simulink model "Rudder_system_control2020_5"  (R2022b)
settings: Solver=VariableStepAuto  StartTime=0.0  StopTime=1800  MaxStep=0.02  RelTol=1e-3  AbsTol=1e-3  EnableMultiTasking=on
model workspace (MAT data in the model file):
  lowerLimitSaturation = -0.1
  upperLimitSaturation = 0.1
values from neighbouring files (symbols this model uses):
  Fg = 1    [start.m]
  H = 1    [start.m]
  Js = 1    [start.m]
  PistonStroke = 0.6    [start.m]
undefined symbols (not defined in the file or in its folder): sigbuilder_block
libraries: fl_lib x71, nesl_utility x16, sh_lib x2, simulink x1, aerolibconvert2 x1
(part 2 of 2)

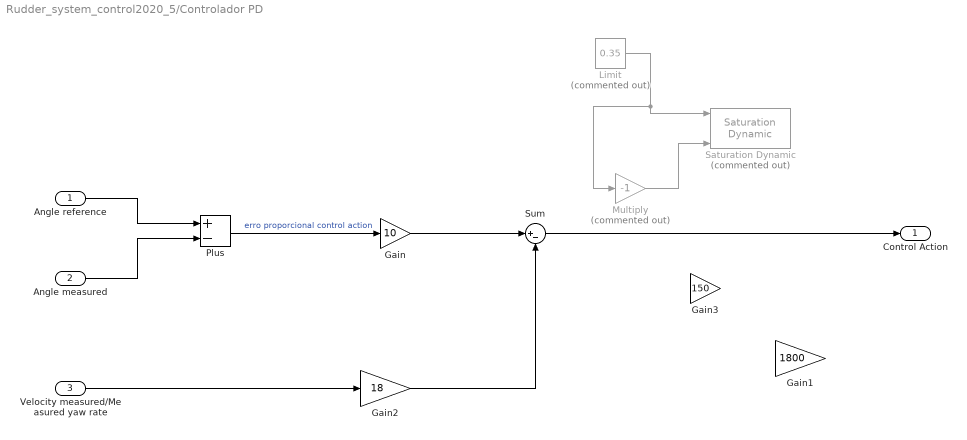
== system Rudder_system_control2020_5/Controlador PD ==
  Angle reference : Inport
  Angle measured : Inport  Port=2
  Velocity measured/Measured yaw rate : Inport  Port=3
  Gain : Gain  Gain=10
  Gain1 : Gain  Gain=1800
  Gain2 : Gain  Gain=18
  Gain3 : Gain  Gain=150
  Limit : Constant  Commented=on  Value=0.35
  Multiply : Gain  Commented=on  Gain=-1
  Plus : Sum  Inputs=+-
  Saturation Dynamic : simulink/Discontinuities/Saturation Dynamic  Commented=on  OutMin=[]  OutMax=[]  OutDataTypeStr=Inherit: Same as second input  OutDataType=fixdt(1, 16)  OutScaling=2^-10  DoSatur=off
  Sum : Sum  Inputs=|+-
  Control Action : Outport
  wires:
  Plus/1 -> Gain/1  "erro proporcional control action"
  Angle reference/1 -> Plus/1
  Angle measured/1 -> Plus/2
  Limit/1 -> Multiply/1, Saturation Dynamic/1
  Multiply/1 -> Saturation Dynamic/3
  Velocity measured/Measured yaw rate/1 -> Gain2/1
  Gain/1 -> Sum/1
  Sum/1 -> Control Action/1
  Gain2/1 -> Sum/2

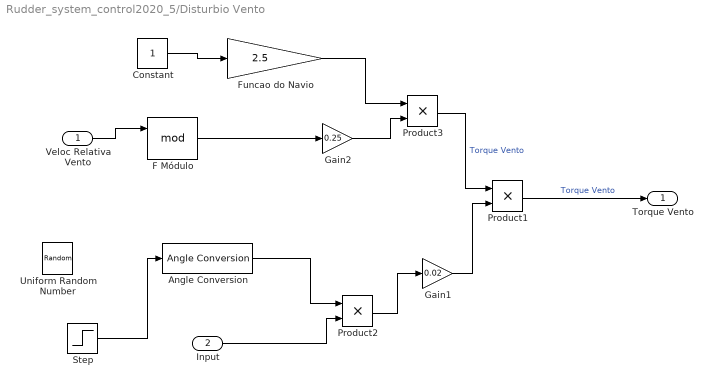
== system Rudder_system_control2020_5/Disturbio Vento ==
  Veloc Relativa Vento : Inport
  Input : Inport  Port=2
  Angle Conversion : aerolibconvert2/Angle Conversion  IU=rad  OU=deg
  Constant : Constant
  F Módulo : Math  Operator=mod
  Funcao do Navio : Gain  Gain=2.5
  Gain1 : Gain  Gain=0.02
  Gain2 : Gain  Gain=0.25
  Product1 : Product
  Product2 : Product
  Product3 : Product
  Step : Step  After=pi*0.5  SampleTime=0
  Uniform Random Number : UniformRandomNumber  Minimum=-2*pi  Maximum=2*pi  SampleTime=30
  Torque Vento : Outport
  wires:
  F Módulo/1 -> Gain2/1
  Gain2/1 -> Product3/2
  Angle Conversion/1 -> Product2/1
  Input/1 -> Product2/2
  Product2/1 -> Gain1/1
  Product1/1 -> Torque Vento/1  "Torque Vento"
  Veloc Relativa Vento/1 -> F Módulo/1
  Funcao do Navio/1 -> Product3/1
  Product3/1 -> Product1/1  "Torque Vento"
  Constant/1 -> Funcao do Navio/1
  Gain1/1 -> Product1/2
  Step/1 -> Angle Conversion/1

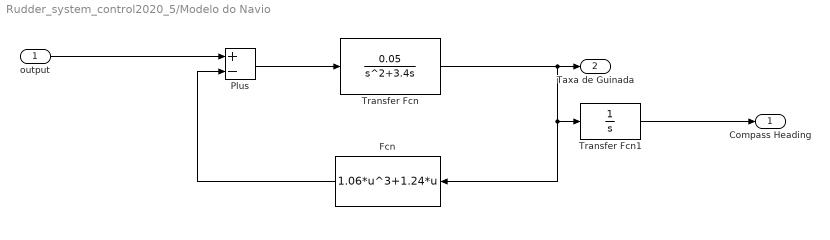
== system Rudder_system_control2020_5/Modelo do Navio ==
  output : Inport
  Fcn : Fcn  Expr=1.06*u^3+1.24*u
  Plus : Sum  Inputs=+-
  Transfer Fcn : TransferFcn  Numerator=[0.05]  Denominator=[1 3.4 0]
  Transfer Fcn1 : TransferFcn  Denominator=[1 0]
  Compass Heading : Outport
  Taxa de Guinada : Outport  Port=2
  wires:
  output/1 -> Plus/1
  Transfer Fcn1/1 -> Compass Heading/1
  Fcn/1 -> Plus/2
  Transfer Fcn/1 -> Fcn/1, Transfer Fcn1/1, Taxa de Guinada/1
  Plus/1 -> Transfer Fcn/1

== system Rudder_system_control2020_5/Signal Builder ==
  Demux : Demux  Tag=STV Demux  Outputs=1
      settings: DisplayOption=none
  FromWs : FromWorkspace  Tag=STV FromWs  VariableName=tuvar
      SigBuilderData=|
      | common.afterFinalStr = 'Extrapolate'
      | common.sampleTime = 0
      | dataSet.timeRange = [0 3000]
      | dataSet.name = 'Group 1'
      | sbobj.Groups.Name = 'Group 1'
      | sbobj.Groups.Signals.Name = 'Signal 2'
      | sbobj.Groups.Signals.XData = [0 10 10 3000]
      | sbobj.Groups.Signals.YData = [0 0 1 1]
      | sbobj.Groups.TimeRange = [0 3000]
  Signal 2 : Outport  Tag=STV Outport
  wires:
  FromWs/1 -> Demux/1
  Demux/1 -> Signal 2/1

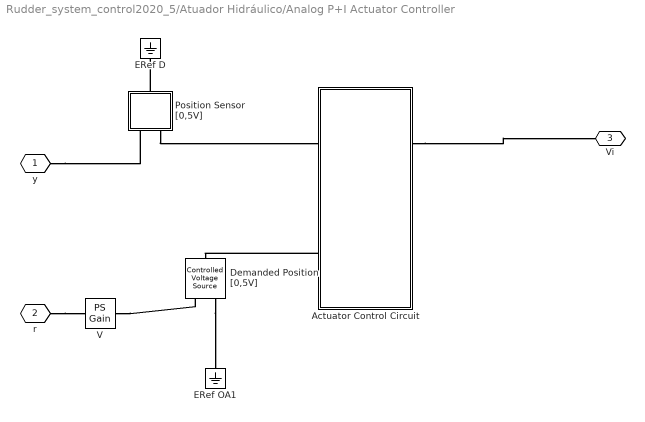
== system Rudder_system_control2020_5/Atuador Hidráulico/Analog P+I Actuator Controller ==
  Actuator Control Circuit : Subsystem  Tag=PublishSubsystem
  Demanded Position [0,5V] : fl_lib/Electrical/Electrical Sources/Controlled Voltage Source
  ERef D : fl_lib/Electrical/Electrical Elements/Electrical Reference
  ERef OA1 : fl_lib/Electrical/Electrical Elements/Electrical Reference
  Position Sensor [0,5V] : Subsystem
  V : fl_lib/Physical Signals/Functions/PS Gain  gain=1 V
  y : PMIOPort  Tag=PMCPort  Side=Left
  r : PMIOPort  Tag=PMCPort  Port=2  Side=Left
  Vi : PMIOPort  Port=3  Side=Right
  connections:
  y/RConn1 -- Position Sensor [0,5V]/LConn1
  r/RConn1 -- V/LConn1
  Actuator Control Circuit/LConn2 -- Demanded Position [0,5V]/LConn1
  Position Sensor [0,5V]/RConn1 -- ERef D/LConn1
  Position Sensor [0,5V]/LConn2 -- Actuator Control Circuit/LConn1
  Actuator Control Circuit/RConn1 -- Vi/RConn1
  Demanded Position [0,5V]/RConn2 -- ERef OA1/LConn1
  V/RConn1 -- Demanded Position [0,5V]/RConn1

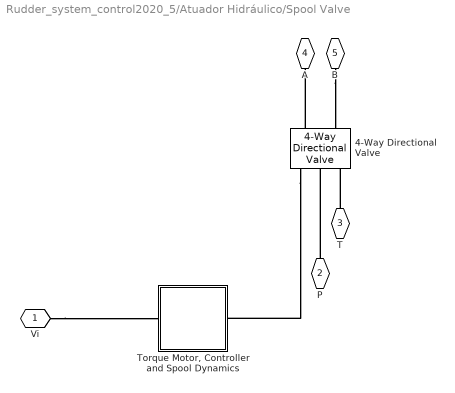
== system Rudder_system_control2020_5/Atuador Hidráulico/Spool Valve ==
  4-Way Directional Valve : sh_lib/Valves/Directional Valves/4-Way Directional Valve  area_spec=sh.valves.directional_valves.enum.area_spec.identical  mdl_type_identical=sh.valves.directional_valves.enum.mdl_type.linear  mdl_type_different=sh.valves.directional_valves.enum.mdl_type.linear  interp_method_identical=sh.valves.directional_valves.enum.interp_method.linear  interp_method_different=sh.valves.directional_valves.enum.interp_method.linear  extrap_method_identical=sh.valves.directional_valves.enum.extrap_method.linear  extrap_method_different=sh.valves.directional_valves.enum.extrap_method.linear  A_leak=1e-12 m^2  C_d=0.7  lam_spec=sh.valves.directional_valves.enum.lam_spec.pressure_ratio  B_lam=0.999  Re_cr=12  opening_max=0.005 m  area_max=0.5e-4 m^2  opening_max_P_A=0.005 m  area_max_P_A=0.5e-4 m^2  opening_max_P_B=0.005 m  area_max_P_B=0.5e-4 m^2  opening_max_A_T=0.005 m  area_max_A_T=0.5e-4 m^2  opening_max_B_T=0.005 m  area_max_B_T=0.5e-4 m^2  opening_area_tab=[-.002, 0, .002, .005, .015] m  area_tab=[1e-09, 2.0352e-07, 4.0736e-05, .00011438, .00034356] m^2  opening_flow_rate_tab=[-.002, 0, .002, .005, .015] m  pressure_tab=[-10000000, -5000000, -2000000, 2000000, 5000000, 10000000] Pa  flow_rate_tab=[-1e-07, -7.0711e-08, -4.4721e-08, 4.4721e-08, 7.0711e-08, 1e-07; -2.0352e-05, -1.4391e-05, -9.1017e-06, 9.1017e-06, 1.4391e-05, 2.0352e-05; -.0040736, -.0028805, -.0018218, .0018218, .0028805, .0040736; -.011438, -.0080879, -.0051152, .0051152, .0080879, .011438; -.034356, -.024293, -.015364, .015364, .024293, .034356] m^3/s  opening_area_tab_P_A=[-.002, 0, .002, .005, .015] m  area_tab_P_A=[1e-09, 2.0352e-07, 4.0736e-05, .00011438, .00034356] m^2  opening_flow_rate_tab_P_A=[-.002, 0, .002, .005, .015] m  pressure_tab_P_A=[-10000000, -5000000, -2000000, 2000000, 5000000, 10000000] Pa  flow_rate_tab_P_A=[-1e-07, -7.0711e-08, -4.4721e-08, 4.4721e-08, 7.0711e-08, 1e-07; -2.0352e-05, -1.4391e-05, -9.1017e-06, 9.1017e-06, 1.4391e-05, 2.0352e-05; -.0040736, -.0028805, -.0018218, .0018218, .0028805, .0040736; -.011438, -.0080879, -.0051152, .0051152, .0080879, .011438; -.034356, -.024293, -.015364, .015364, .024293, .034356] m^3/s  opening_area_tab_P_B=[-.002, 0, .002, .005, .015] m  area_tab_P_B=[1e-09, 2.0352e-07, 4.0736e-05, .00011438, .00034356] m^2  opening_flow_rate_tab_P_B=[-.002, 0, .002, .005, .015] m  pressure_tab_P_B=[-10000000, -5000000, -2000000, 2000000, 5000000, 10000000] Pa  flow_rate_tab_P_B=[-1e-07, -7.0711e-08, -4.4721e-08, 4.4721e-08, 7.0711e-08, 1e-07; -2.0352e-05, -1.4391e-05, -9.1017e-06, 9.1017e-06, 1.4391e-05, 2.0352e-05; -.0040736, -.0028805, -.0018218, .0018218, .0028805, .0040736; -.011438, -.0080879, -.0051152, .0051152, .0080879, .011438; -.034356, -.024293, -.015364, .015364, .024293, .034356] m^3/s  opening_area_tab_A_T=[-.002, 0, .002, .005, .015] m  area_tab_A_T=[1e-09, 2.0352e-07, 4.0736e-05, .00011438, .00034356] m^2  opening_flow_rate_tab_A_T=[-.002, 0, .002, .005, .015] m  pressure_tab_A_T=[-10000000, -5000000, -2000000, 2000000, 5000000, 10000000] Pa  flow_rate_tab_A_T=[-1e-07, -7.0711e-08, -4.4721e-08, 4.4721e-08, 7.0711e-08, 1e-07; -2.0352e-05, -1.4391e-05, -9.1017e-06, 9.1017e-06, 1.4391e-05, 2.0352e-05; -.0040736, -.0028805, -.0018218, .0018218, .0028805, .0040736; -.011438, -.0080879, -.0051152, .0051152, .0080879, .011438; -.034356, -.024293, -.015364, .015364, .024293, .034356] m^3/s  opening_area_tab_B_T=[-.002, 0, .002, .005, .015] m  area_tab_B_T=[1e-09, 2.0352e-07, 4.0736e-05, .00011438, .00034356] m^2  opening_flow_rate_tab_B_T=[-.002, 0, .002, .005, .015] m  pressure_tab_B_T=[-10000000, -5000000, -2000000, 2000000, 5000000, 10000000] Pa  flow_rate_tab_B_T=[-1e-07, -7.0711e-08, -4.4721e-08, 4.4721e-08, 7.0711e-08, 1e-07; -2.0352e-05, -1.4391e-05, -9.1017e-06, 9.1017e-06, 1.4391e-05, 2.0352e-05; -.0040736, -.0028805, -.0018218, .0018218, .0028805, .0040736; -.011438, -.0080879, -.0051152, .0051152, .0080879, .011438; -.034356, -.024293, -.015364, .015364, .024293, .034356] m^3/s  x_0_P_A=0 m  x_0_P_B=0 m  x_0_A_T=0 m  x_0_B_T=0 m
      settings: InternalSimscapePortConfiguration="{\"Bottom\":[],\"Left\":[{\"id\":\"A\",\"label\":\"A\",\"type\":\"foundation.hydraulic.hydraulic\"},{\"id\":\"B\",\"label\":\"B\",\"type\":\"foundation.hydraulic.hydraulic\"}],\"Right\":[{\"id\":\"S\",\"label\":\"S\",\"type\":\"input\"},{\"id\":\"P\",\"label\":\"P\",\"type\":\"foundation.hydraulic.hydraulic\"},{\"id\":\"T\",\"label\":\"T\",\"type\":\"foundation.hydraulic.hydraulic\"}],\"Top\":[]}"
  "Torque Motor, Controller and Spool Dynamics" : Subsystem
  Vi : PMIOPort  Tag=PMCPort  Side=Left
  P : PMIOPort  Tag=PMCPort  Port=2  Side=Left
  T : PMIOPort  Tag=PMCPort  Port=3  Side=Left
  A : PMIOPort  Tag=PMCPort  Port=4  Side=Right
  B : PMIOPort  Tag=PMCPort  Port=5  Side=Right
  connections:
  Vi/RConn1 -- "Torque Motor, Controller and Spool Dynamics"/LConn1
  4-Way Directional Valve/RConn1 -- "Torque Motor, Controller and Spool Dynamics"/RConn1
  4-Way Directional Valve/LConn1 -- A/RConn1
  B/RConn1 -- 4-Way Directional Valve/LConn2
  P/RConn1 -- 4-Way Directional Valve/RConn2
  T/RConn1 -- 4-Way Directional Valve/RConn3

== system Rudder_system_control2020_5/Atuador Hidráulico/Supply Pressure ==
  Supply Pressure : Constant  Value=200
  bar : nesl_utility/Simulink-PS Converter  PhysicalDomain=network_engine_domain  SubClassName=ps_input  LeftPortType=input  RightPortType=output  PseudoPeriodic=off  Frequencies=[]  NoiseDistribution=none  NoiseParameters=[]  Unit=bar  AffineConversion=off  FilteringAndDerivatives=zero  SimscapeFilterOrder=1  InputFilterTimeConstant=.001  UdotUserProvided=0
  S : PMIOPort  Side=Right
  wires:
  Supply Pressure/1 -> bar/1
  connections:
  bar/RConn1 -- S/RConn1

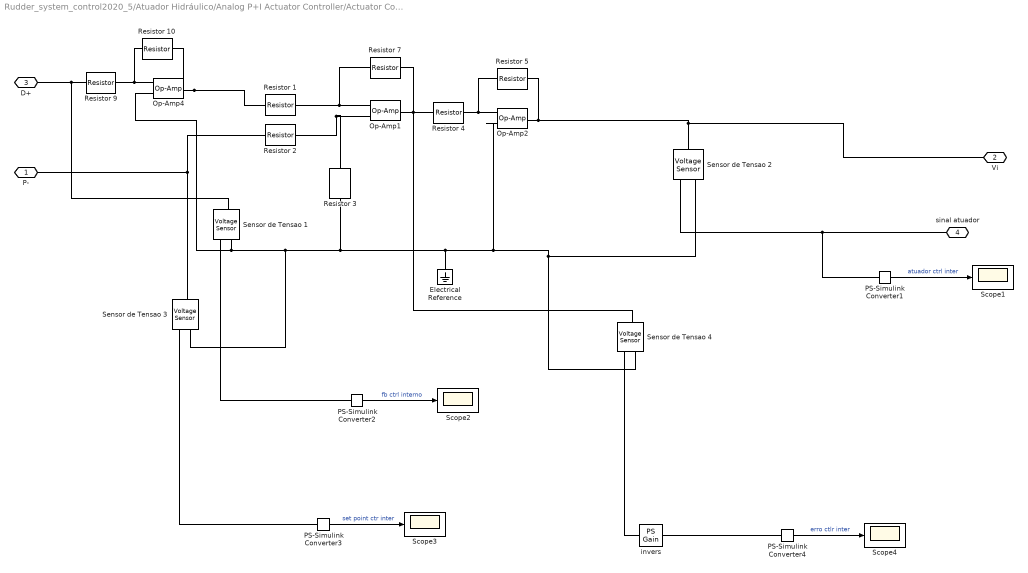
== system Rudder_system_control2020_5/Atuador Hidráulico/Analog P+I Actuator Controller/Actuator Control Circuit ==
  Electrical Reference : fl_lib/Electrical/Electrical Elements/Electrical Reference
  Op-Amp1 : fl_lib/Electrical/Electrical Elements/Op-Amp  outI_specify=off  outI_priority=None  outI=0 A  outI_nominal_specify=off  outI_nominal_unit=A  outI_nominal_value=1
  Op-Amp2 : fl_lib/Electrical/Electrical Elements/Op-Amp  outI_specify=off  outI_priority=None  outI=0 A  outI_nominal_specify=off  outI_nominal_unit=A  outI_nominal_value=1
  Op-Amp4 : fl_lib/Electrical/Electrical Elements/Op-Amp  outI_specify=off  outI_priority=None  outI=0 A  outI_nominal_specify=off  outI_nominal_unit=A  outI_nominal_value=1
  PS-Simulink Converter{1..4} (4 alike) : nesl_utility/PS-Simulink Converter  PhysicalDomain=network_engine_domain  SubClassName=ps_output  LeftPortType=input  RightPortType=output  PseudoPeriodic=off  Frequencies=[]  VectorFormat=1-D array  Unit=inherit  AffineConversion=off
  Resistor {1..3,7,9..10} (6 alike) : fl_lib/Electrical/Electrical Elements/Resistor  R=1 Ohm  i_specify=off  i_priority=None  i=0 A  i_nominal_specify=off  i_nominal_unit=A  i_nominal_value=1  v_specify=off  v_priority=None  v=0 V  v_nominal_specify=off  v_nominal_unit=V  v_nominal_value=1
  Resistor 4 : fl_lib/Electrical/Electrical Elements/Resistor  R=100 Ohm  i_specify=off  i_priority=None  i=0 A  i_nominal_specify=off  i_nominal_unit=A  i_nominal_value=1  v_specify=off  v_priority=None  v=0 V  v_nominal_specify=off  v_nominal_unit=V  v_nominal_value=1
  Resistor 5 : fl_lib/Electrical/Electrical Elements/Resistor  R=910 Ohm  i_specify=off  i_priority=None  i=0 A  i_nominal_specify=off  i_nominal_unit=A  i_nominal_value=1  v_specify=off  v_priority=None  v=0 V  v_nominal_specify=off  v_nominal_unit=V  v_nominal_value=1
  Scope{1..4} (4 alike) : Scope
  Sensor de Tensao {1..4} (4 alike) : fl_lib/Electrical/Electrical Sensors/Voltage Sensor
  invers : fl_lib/Physical Signals/Functions/PS Gain  gain=-1
  P- : PMIOPort  Side=Left
  Vi : PMIOPort  Port=2  Side=Right
  D+ : PMIOPort  Port=3  Side=Left
  sinal atuador : PMIOPort  Port=4  Side=Right
  wires:
  PS-Simulink Converter1/1 -> Scope1/1  "atuador ctrl inter"
  PS-Simulink Converter2/1 -> Scope2/1  "fb ctrl interno"
  PS-Simulink Converter3/1 -> Scope3/1  "set point ctr inter"
  PS-Simulink Converter4/1 -> Scope4/1  "erro ctlr inter"
  connections:
  D+/RConn1 -- Sensor de Tensao 1/LConn1 -- Resistor 9/LConn1
  Resistor 9/RConn1 -- Resistor 10/LConn1 -- Op-Amp4/LConn2
  Op-Amp1/RConn1 -- Resistor 7/RConn1 -- Sensor de Tensao 4/LConn1 -- Resistor 4/LConn1
  Resistor 2/RConn1 -- Op-Amp1/LConn1 -- Resistor 3/LConn1
  Op-Amp4/LConn1 -- Sensor de Tensao 1/RConn2 -- Sensor de Tensao 3/RConn2 -- Resistor 3/RConn1 -- Electrical Reference/LConn1 -- Sensor de Tensao 2/RConn2 -- Sensor de Tensao 4/RConn2 -- Op-Amp2/LConn1
  Resistor 5/LConn1 -- Op-Amp2/LConn2 -- Resistor 4/RConn1
  Op-Amp1/LConn2 -- Resistor 7/LConn1 -- Resistor 1/RConn1
  Sensor de Tensao 2/RConn1 -- PS-Simulink Converter1/LConn1 -- sinal atuador/RConn1
  Op-Amp4/RConn1 -- Resistor 10/RConn1 -- Resistor 1/LConn1
  Sensor de Tensao 3/LConn1 -- P-/RConn1 -- Resistor 2/LConn1
  Sensor de Tensao 1/RConn1 -- PS-Simulink Converter2/LConn1
  Sensor de Tensao 3/RConn1 -- PS-Simulink Converter3/LConn1
  Op-Amp2/RConn1 -- Vi/RConn1 -- Sensor de Tensao 2/LConn1 -- Resistor 5/RConn1
  invers/RConn1 -- PS-Simulink Converter4/LConn1
  invers/LConn1 -- Sensor de Tensao 4/RConn1

== system Rudder_system_control2020_5/Atuador Hidráulico/Analog P+I Actuator Controller/Position Sensor [0,5V] ==
  Controlled Voltage Source : fl_lib/Electrical/Electrical Sources/Controlled Voltage Source
  + : PMIOPort  Side=Right
  y : PMIOPort  Port=2  Side=Left
  - : PMIOPort  Port=3  Side=Left
  connections:
  +/RConn1 -- Controlled Voltage Source/LConn1
  -/RConn1 -- Controlled Voltage Source/RConn2
  Controlled Voltage Source/RConn1 -- y/RConn1

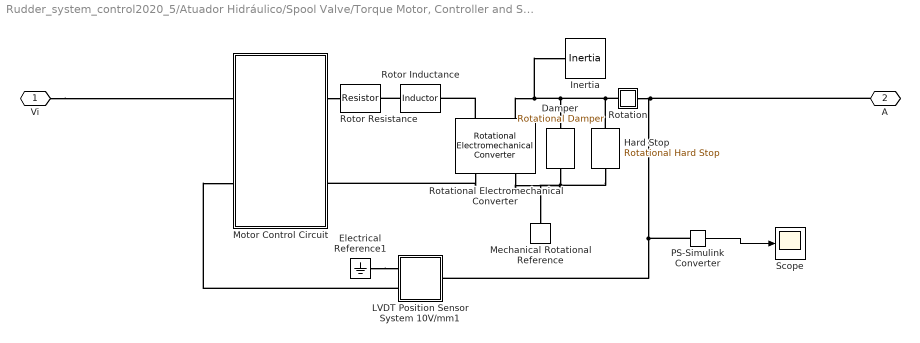
== system Rudder_system_control2020_5/Atuador Hidráulico/Spool Valve/Torque Motor, Controller and Spool Dynamics ==
  Damper : fl_lib/Mechanical/Rotational Elements/Rotational Damper  D=lambda N*m/(rad/s)  w_specify=off  w_priority=High  w=0 rad/s  w_nominal_specify=off  w_nominal_unit=rad/s  w_nominal_value=1  t_specify=off  t_priority=High  t=0 N*m  t_nominal_specify=off  t_nominal_unit=N*m  t_nominal_value=1
  Electrical Reference1 : fl_lib/Electrical/Electrical Elements/Electrical Reference
  Hard Stop : fl_lib/Mechanical/Rotational Elements/Rotational Hard Stop  upper_bnd=x_max*1e-3/G rad  lower_bnd=-x_max*1e-3/G rad  stiff_up=1e+06 N*m/rad  stiff_low=1e+6 N*m/rad  D_up=0.05 N*m/(rad/s)  D_low=0.05 N*m/(rad/s)  model=3  transition=0.001 rad  w_specify=off  w_priority=High  w=0 rad/s  w_nominal_specify=off  w_nominal_unit=rad/s  w_nominal_value=1  t_specify=off  t_priority=High  t=0 N*m  t_nominal_specify=off  t_nominal_unit=N*m  t_nominal_value=1  phi_specify=on  phi_priority=High  phi=0 rad  phi_nominal_specify=off  phi_nominal_unit=rad  phi_nominal_value=1
  Inertia : fl_lib/Mechanical/Rotational Elements/Inertia  inertia=J kg*m^2  num_ports=foundation.enum.numPorts2.one  w_specify=off  w_priority=High  w=0 rad/s  w_nominal_specify=off  w_nominal_unit=rad/s  w_nominal_value=1  t_specify=off  t_priority=High  t=0 N*m  t_nominal_specify=off  t_nominal_unit=N*m  t_nominal_value=1
  LVDT Position Sensor System 10V/mm1 : Subsystem
  Mechanical Rotational Reference : fl_lib/Mechanical/Rotational Elements/Mechanical Rotational Reference
  Motor Control Circuit : Subsystem  Tag=PublishSubsystem
  PS-Simulink Converter : nesl_utility/PS-Simulink Converter  PhysicalDomain=network_engine_domain  SubClassName=ps_output  LeftPortType=input  RightPortType=output  PseudoPeriodic=off  Frequencies=[]  VectorFormat=1-D array  Unit=inherit  AffineConversion=off
  Rotation : Subsystem
      mask Display: disp('A')
  Rotational Electromechanical Converter : fl_lib/Electrical/Electrical Elements/Rotational Electromechanical Converter  K=Kt V/(rad/s)  i_specify=off  i_priority=High  i=0 A  i_nominal_specify=off  i_nominal_unit=A  i_nominal_value=1  v_specify=off  v_priority=High  v=0 V  v_nominal_specify=off  v_nominal_unit=V  v_nominal_value=1  t_specify=off  t_priority=High  t=0 N*m  t_nominal_specify=off  t_nominal_unit=N*m  t_nominal_value=1  w_specify=off  w_priority=High  w=0 rad/s  w_nominal_specify=off  w_nominal_unit=rad/s  w_nominal_value=1
  Rotor Inductance : fl_lib/Electrical/Electrical Elements/Inductor  l=L H  r=0 Ohm  g=1e-09 1/Ohm  i_specify=off  i_priority=High  i=0 A  i_nominal_specify=off  i_nominal_unit=A  i_nominal_value=1  v_specify=off  v_priority=High  v=0 V  v_nominal_specify=off  v_nominal_unit=V  v_nominal_value=1  i_L_specify=on  i_L_priority=High  i_L=0 A  i_L_nominal_specify=off  i_L_nominal_unit=A  i_L_nominal_value=1
  Rotor Resistance : fl_lib/Electrical/Electrical Elements/Resistor  Tag=Factory Generic  R=R Ohm  i_specify=off  i_priority=High  i=0 A  i_nominal_specify=off  i_nominal_unit=A  i_nominal_value=1  v_specify=off  v_priority=High  v=0 V  v_nominal_specify=off  v_nominal_unit=V  v_nominal_value=1
  Scope : Scope
  Vi : PMIOPort  Side=Left
  A : PMIOPort  Port=2  Side=Right
  wires:
  PS-Simulink Converter/1 -> Scope/1
  connections:
  Damper/RConn1 -- Hard Stop/RConn1 -- Rotational Electromechanical Converter/RConn2 -- Mechanical Rotational Reference/LConn1
  Rotational Electromechanical Converter/LConn1 -- Rotor Inductance/RConn1
  Rotor Inductance/LConn1 -- Rotor Resistance/RConn1
  Motor Control Circuit/RConn1 -- Rotor Resistance/LConn1
  Vi/RConn1 -- Motor Control Circuit/LConn1
  LVDT Position Sensor System 10V/mm1/RConn2 -- Motor Control Circuit/LConn2
  Rotational Electromechanical Converter/RConn1 -- Motor Control Circuit/RConn2
  Electrical Reference1/LConn1 -- LVDT Position Sensor System 10V/mm1/RConn1
  A/RConn1 -- Rotation/RConn1 -- PS-Simulink Converter/LConn1 -- LVDT Position Sensor System 10V/mm1/LConn1
  Hard Stop/LConn1 -- Rotation/LConn1 -- Rotational Electromechanical Converter/LConn2 -- Inertia/LConn1 -- Damper/LConn1

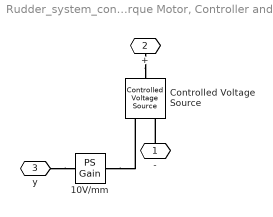
== system Rudder_system_control2020_5/Atuador Hidráulico/Spool Valve/Torque Motor, Controller and Spool Dynamics/LVDT Position Sensor System 10V//mm1 ==
  10V/mm : fl_lib/Physical Signals/Functions/PS Gain  gain=10 V/mm
  Controlled Voltage Source : fl_lib/Electrical/Electrical Sources/Controlled Voltage Source
  - : PMIOPort  Side=Right
  + : PMIOPort  Port=2  Side=Right
  y : PMIOPort  Port=3  Side=Left
  connections:
  y/RConn1 -- 10V/mm/LConn1
  -/RConn1 -- Controlled Voltage Source/RConn2
  +/RConn1 -- Controlled Voltage Source/LConn1
  10V/mm/RConn1 -- Controlled Voltage Source/RConn1

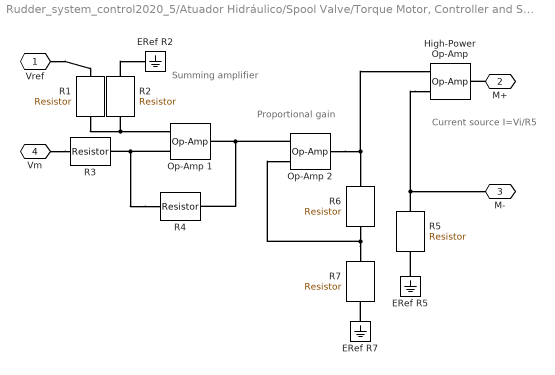
== system Rudder_system_control2020_5/Atuador Hidráulico/Spool Valve/Torque Motor, Controller and Spool Dynamics/Motor Control Circuit ==
  note: Current source
      | I=Vi/R5
  note: Summing
      | amplifier
  note: Proportional gain
  ERef R2 : fl_lib/Electrical/Electrical Elements/Electrical Reference
  ERef R5 : fl_lib/Electrical/Electrical Elements/Electrical Reference
  ERef R7 : fl_lib/Electrical/Electrical Elements/Electrical Reference
  High-Power Op-Amp : fl_lib/Electrical/Electrical Elements/Op-Amp  outI_specify=off  outI_priority=High  outI=0 A  outI_nominal_specify=off  outI_nominal_unit=A  outI_nominal_value=1
  Op-Amp 1 : fl_lib/Electrical/Electrical Elements/Op-Amp  outI_specify=off  outI_priority=High  outI=0 A  outI_nominal_specify=off  outI_nominal_unit=A  outI_nominal_value=1
  Op-Amp 2 : fl_lib/Electrical/Electrical Elements/Op-Amp  outI_specify=off  outI_priority=High  outI=0 A  outI_nominal_specify=off  outI_nominal_unit=A  outI_nominal_value=1
  R1 : fl_lib/Electrical/Electrical Elements/Resistor  R=R_controller(1) Ohm  i_specify=off  i_priority=High  i=0 A  i_nominal_specify=off  i_nominal_unit=A  i_nominal_value=1  v_specify=off  v_priority=High  v=0 V  v_nominal_specify=off  v_nominal_unit=V  v_nominal_value=1
  R2 : fl_lib/Electrical/Electrical Elements/Resistor  R=R_controller(2) Ohm  i_specify=off  i_priority=High  i=0 A  i_nominal_specify=off  i_nominal_unit=A  i_nominal_value=1  v_specify=off  v_priority=High  v=0 V  v_nominal_specify=off  v_nominal_unit=V  v_nominal_value=1
  R3 : fl_lib/Electrical/Electrical Elements/Resistor  R=R_controller(3) Ohm  i_specify=off  i_priority=High  i=0 A  i_nominal_specify=off  i_nominal_unit=A  i_nominal_value=1  v_specify=off  v_priority=High  v=0 V  v_nominal_specify=off  v_nominal_unit=V  v_nominal_value=1
  R4 : fl_lib/Electrical/Electrical Elements/Resistor  R=R_controller(4) Ohm  i_specify=off  i_priority=High  i=0 A  i_nominal_specify=off  i_nominal_unit=A  i_nominal_value=1  v_specify=off  v_priority=High  v=0 V  v_nominal_specify=off  v_nominal_unit=V  v_nominal_value=1
  R5 : fl_lib/Electrical/Electrical Elements/Resistor  R=R_controller(5) Ohm  i_specify=off  i_priority=High  i=0 A  i_nominal_specify=off  i_nominal_unit=A  i_nominal_value=1  v_specify=off  v_priority=High  v=0 V  v_nominal_specify=off  v_nominal_unit=V  v_nominal_value=1
  R6 : fl_lib/Electrical/Electrical Elements/Resistor  R=R_controller(6) Ohm  i_specify=off  i_priority=High  i=0 A  i_nominal_specify=off  i_nominal_unit=A  i_nominal_value=1  v_specify=off  v_priority=High  v=0 V  v_nominal_specify=off  v_nominal_unit=V  v_nominal_value=1
  R7 : fl_lib/Electrical/Electrical Elements/Resistor  R=R_controller(7) Ohm  i_specify=off  i_priority=High  i=0 A  i_nominal_specify=off  i_nominal_unit=A  i_nominal_value=1  v_specify=off  v_priority=High  v=0 V  v_nominal_specify=off  v_nominal_unit=V  v_nominal_value=1
  Vref : PMIOPort  Side=Left
  M+ : PMIOPort  Port=2  Side=Right
  M- : PMIOPort  Port=3  Side=Right
  Vm : PMIOPort  Port=4  Side=Left
  connections:
  ERef R7/LConn1 -- R7/RConn1
  R2/RConn1 -- ERef R2/LConn1
  ERef R5/LConn1 -- R5/RConn1
  Op-Amp 2/RConn1 -- High-Power Op-Amp/LConn1 -- R6/LConn1
  High-Power Op-Amp/LConn2 -- M-/RConn1 -- R5/LConn1
  R2/LConn1 -- Op-Amp 1/LConn1 -- R1/RConn1
  R4/LConn1 -- Op-Amp 1/LConn2 -- R3/RConn1
  Op-Amp 2/LConn1 -- Op-Amp 1/RConn1 -- R4/RConn1
  R7/LConn1 -- Op-Amp 2/LConn2 -- R6/RConn1
  Vref/RConn1 -- R1/LConn1
  M+/RConn1 -- High-Power Op-Amp/RConn1
  Vm/RConn1 -- R3/LConn1

== system Rudder_system_control2020_5/Atuador Hidráulico/Spool Valve/Torque Motor, Controller and Spool Dynamics/Rotation ==
  Displacement : fl_lib/Physical Signals/Functions/PS Gain  gain=G m/rad
  Ideal Rotational Motion Sensor : fl_lib/Mechanical/Mechanical Sensors/Ideal Rotational Motion Sensor  reference=foundation.enum.MeasurementReference.difference  acceleration_port=false  velocity_port=true  position_port=true  wrap_angle=simscape.enum.onoff.off  offset=0 rad
  Mechanical Rotational Reference1 : fl_lib/Mechanical/Rotational Elements/Mechanical Rotational Reference
  R : PMIOPort  Side=Left
  A : PMIOPort  Port=2  Side=Right
  connections:
  Mechanical Rotational Reference1/LConn1 -- Ideal Rotational Motion Sensor/RConn1
  Ideal Rotational Motion Sensor/RConn3 -- Displacement/LConn1
  Displacement/RConn1 -- A/RConn1
  Ideal Rotational Motion Sensor/LConn1 -- R/RConn1
